simulink model "MCity_cs"  (Simulink 8.9)
settings: Solver=ode5  StartTime=0.0  StopTime=2.95  FixedStep=1/200  RelTol=1e-3
PreLoadFcn:
  | check_NUTS_defined;
  | 
  | assignin('base',['model_closed_' bdroot],false);
InitFcn:
  | PreScanExperimentInitFcn(bdroot)
StopFcn:
  | PreScanExperimentStopFcn(bdroot)
values from neighbouring files (symbols this model uses):
  d_offset = -18.15    [monocityTestLeftTurn.mat]    (also in simulation_leftTurn_PreScan.m = dl/vl*vh - 43 + R)
undefined symbols (not defined in the file or in its folder): DiscIntNeverNeededParam, warningInitialVelocity, x0
libraries: simulink x73, PreScanSimulinkLibrary x14, simulink_extras x10, PreScanUsefulBlocks x4
(part 4 of 11)

== system MCity_cs/TrafficLightDoubleUS_1/Traffic_Light On/Off  ==
  Range : Inport
  Compare To Constant : simulink/Logic and Bit Operations/Compare To Constant  relop=>=  const=1  OutDataTypeStr=uint8
  Constant : Constant
  Constant1 : Constant  Value=0
  Data Type Conversion{1,3..5} (4 alike) : DataTypeConversion
  Delay : Delay  DelayLength=40
  Logical Operator : Logic  Operator=NOT  AllPortsSameDT=off  OutDataTypeStr=boolean
  Logical Operator1 : Logic  Operator=NOT  AllPortsSameDT=off  OutDataTypeStr=boolean
  Logical Operator2 : Logic  Operator=NOT  AllPortsSameDT=off  OutDataTypeStr=boolean
  Logical Operator3 : Logic  AllPortsSameDT=off  OutDataTypeStr=boolean
  Logical Operator4 : Logic  AllPortsSameDT=off  OutDataTypeStr=boolean
  MinMax : MinMax  Function=max
  Pulse Generator : DiscretePulseGenerator  PulseType=Time based  Period=10  PulseWidth=50
  Switch{,1..3} (4 alike) : Switch  Criteria=u2 > Threshold
  Red : Outport
  Orange : Outport  Port=2
  Green : Outport  Port=3
  wires:
  Pulse Generator/1 -> Logical Operator1/1, Switch2/3
  Logical Operator1/1 -> Delay/1, Logical Operator3/2, Logical Operator4/1
  Delay/1 -> Logical Operator2/1, Logical Operator4/2
  Logical Operator2/1 -> Logical Operator3/1
  Logical Operator3/1 -> Data Type Conversion5/1
  Logical Operator4/1 -> Data Type Conversion4/1
  Constant/1 -> Switch/1
  Compare To Constant/1 -> Switch/2
  Constant1/1 -> Switch/3
  Switch/1 -> MinMax/1
  Logical Operator/1 -> Data Type Conversion3/1, Data Type Conversion1/1
  MinMax/1 -> Logical Operator/1, Switch1/2, Switch3/2, Switch2/1, Switch2/2
  Data Type Conversion1/1 -> Switch1/1
  Data Type Conversion4/1 -> Switch1/3
  Switch1/1 -> Red/1
  Data Type Conversion3/1 -> Switch3/1
  Switch3/1 -> Orange/1
  Data Type Conversion5/1 -> Switch3/3
  Switch2/1 -> Green/1
  Range/1 -> Compare To Constant/1

== system MCity_cs/TrafficLightDoubleUS_1/VISUCasingLights_1_Mux ==
  Red [-] : Inport
  Orange [-] : Inport  Port=2
  Green [-] : Inport  Port=3
  Mux1 : Mux  Inputs=3
  CasingLights : Outport
  wires:
  Green [-]/1 -> Mux1/3
  Mux1/1 -> CasingLights/1
  Orange [-]/1 -> Mux1/2
  Red [-]/1 -> Mux1/1

== system MCity_cs/TrafficLightDoubleUS_1/VISUCasingLights_2_Mux ==
  Red [-] : Inport
  Orange [-] : Inport  Port=2
  Green [-] : Inport  Port=3
  Mux1 : Mux  Inputs=3
  CasingLights : Outport
  wires:
  Green [-]/1 -> Mux1/3
  Mux1/1 -> CasingLights/1
  Orange [-]/1 -> Mux1/2
  Red [-]/1 -> Mux1/1

== system MCity_cs/TrafficLightDoubleUS_10/Perpendicular ==
  Compare To Constant : simulink/Logic and Bit Operations/Compare To Constant  relop=>=  const=1  OutDataTypeStr=uint8
  Constant : Constant
  Constant1 : Constant  Value=0
  Data Type Conversion{1,3..5} (4 alike) : DataTypeConversion
  Delay : Delay  DelayLength=40
  Ground_1 : Ground
  Logical Operator{,1..2,5} (4 alike) : Logic  Operator=NOT  AllPortsSameDT=off  OutDataTypeStr=boolean
  Logical Operator3 : Logic  AllPortsSameDT=off  OutDataTypeStr=boolean
  Logical Operator4 : Logic  AllPortsSameDT=off  OutDataTypeStr=boolean
  MinMax : MinMax  Function=max
  Pulse Generator : DiscretePulseGenerator  PulseType=Time based  Period=10  PulseWidth=50
  Switch{,1..3} (4 alike) : Switch  Criteria=u2 > Threshold
  Red : Outport
  Orange : Outport  Port=2
  Green : Outport  Port=3
  wires:
  Pulse Generator/1 -> Logical Operator5/1
  Logical Operator1/1 -> Delay/1, Logical Operator3/2, Logical Operator4/1
  Delay/1 -> Logical Operator2/1, Logical Operator4/2
  Logical Operator2/1 -> Logical Operator3/1
  Logical Operator3/1 -> Data Type Conversion5/1
  Logical Operator4/1 -> Data Type Conversion4/1
  Constant/1 -> Switch/1
  Compare To Constant/1 -> Switch/2
  Constant1/1 -> Switch/3
  Switch/1 -> MinMax/1
  Logical Operator/1 -> Data Type Conversion3/1, Data Type Conversion1/1
  MinMax/1 -> Logical Operator/1, Switch1/2, Switch3/2, Switch2/1, Switch2/2
  Data Type Conversion1/1 -> Switch1/1
  Data Type Conversion4/1 -> Switch1/3
  Switch1/1 -> Red/1
  Data Type Conversion3/1 -> Switch3/1
  Switch3/1 -> Orange/1
  Data Type Conversion5/1 -> Switch3/3
  Switch2/1 -> Green/1
  Logical Operator5/1 -> Logical Operator1/1, Switch2/3
  Ground_1/1 -> Compare To Constant/1

== system MCity_cs/TrafficLightDoubleUS_10/VISUCasingLights_1_Mux ==
  Red [-] : Inport
  Orange [-] : Inport  Port=2
  Green [-] : Inport  Port=3
  Mux1 : Mux  Inputs=3
  CasingLights : Outport
  wires:
  Green [-]/1 -> Mux1/3
  Mux1/1 -> CasingLights/1
  Orange [-]/1 -> Mux1/2
  Red [-]/1 -> Mux1/1

== system MCity_cs/TrafficLightDoubleUS_10/VISUCasingLights_2_Mux ==
  Red [-] : Inport
  Orange [-] : Inport  Port=2
  Green [-] : Inport  Port=3
  Mux1 : Mux  Inputs=3
  CasingLights : Outport
  wires:
  Green [-]/1 -> Mux1/3
  Mux1/1 -> CasingLights/1
  Orange [-]/1 -> Mux1/2
  Red [-]/1 -> Mux1/1

== system MCity_cs/TrafficLightDoubleUS_2/Traffic_Light On/Off  ==
  Range : Inport
  Compare To Constant : simulink/Logic and Bit Operations/Compare To Constant  relop=>=  const=1  OutDataTypeStr=uint8
  Constant : Constant
  Constant1 : Constant  Value=0
  Data Type Conversion{1,3..5} (4 alike) : DataTypeConversion
  Delay : Delay  DelayLength=40
  Logical Operator : Logic  Operator=NOT  AllPortsSameDT=off  OutDataTypeStr=boolean
  Logical Operator1 : Logic  Operator=NOT  AllPortsSameDT=off  OutDataTypeStr=boolean
  Logical Operator2 : Logic  Operator=NOT  AllPortsSameDT=off  OutDataTypeStr=boolean
  Logical Operator3 : Logic  AllPortsSameDT=off  OutDataTypeStr=boolean
  Logical Operator4 : Logic  AllPortsSameDT=off  OutDataTypeStr=boolean
  MinMax : MinMax  Function=max
  Pulse Generator : DiscretePulseGenerator  PulseType=Time based  Period=10  PulseWidth=50
  Switch{,1..3} (4 alike) : Switch  Criteria=u2 > Threshold
  Red : Outport
  Orange : Outport  Port=2
  Green : Outport  Port=3
  wires:
  Pulse Generator/1 -> Logical Operator1/1, Switch2/3
  Logical Operator1/1 -> Delay/1, Logical Operator3/2, Logical Operator4/1
  Delay/1 -> Logical Operator2/1, Logical Operator4/2
  Logical Operator2/1 -> Logical Operator3/1
  Logical Operator3/1 -> Data Type Conversion5/1
  Logical Operator4/1 -> Data Type Conversion4/1
  Constant/1 -> Switch/1
  Compare To Constant/1 -> Switch/2
  Constant1/1 -> Switch/3
  Switch/1 -> MinMax/1
  Logical Operator/1 -> Data Type Conversion3/1, Data Type Conversion1/1
  MinMax/1 -> Logical Operator/1, Switch1/2, Switch3/2, Switch2/1, Switch2/2
  Data Type Conversion1/1 -> Switch1/1
  Data Type Conversion4/1 -> Switch1/3
  Switch1/1 -> Red/1
  Data Type Conversion3/1 -> Switch3/1
  Switch3/1 -> Orange/1
  Data Type Conversion5/1 -> Switch3/3
  Switch2/1 -> Green/1
  Range/1 -> Compare To Constant/1

== system MCity_cs/TrafficLightDoubleUS_2/VISUCasingLights_1_Mux ==
  Red [-] : Inport
  Orange [-] : Inport  Port=2
  Green [-] : Inport  Port=3
  Mux1 : Mux  Inputs=3
  CasingLights : Outport
  wires:
  Green [-]/1 -> Mux1/3
  Mux1/1 -> CasingLights/1
  Orange [-]/1 -> Mux1/2
  Red [-]/1 -> Mux1/1

== system MCity_cs/TrafficLightDoubleUS_2/VISUCasingLights_2_Mux ==
  Red [-] : Inport
  Orange [-] : Inport  Port=2
  Green [-] : Inport  Port=3
  Mux1 : Mux  Inputs=3
  CasingLights : Outport
  wires:
  Green [-]/1 -> Mux1/3
  Mux1/1 -> CasingLights/1
  Orange [-]/1 -> Mux1/2
  Red [-]/1 -> Mux1/1

== system MCity_cs/TrafficLightDoubleUS_3/Perpendicular ==
  Compare To Constant : simulink/Logic and Bit Operations/Compare To Constant  relop=>=  const=1  OutDataTypeStr=uint8
  Constant : Constant
  Constant1 : Constant  Value=0
  Constant2 : Constant  Value=0
  Data Type Conversion{1,3..5} (4 alike) : DataTypeConversion
  Delay : Delay  DelayLength=40
  Ground_1 : Ground
  Ground_2 : Ground
  Logical Operator : Logic  Operator=NOT  AllPortsSameDT=off  OutDataTypeStr=boolean
  Logical Operator1 : Logic  Operator=NOT  AllPortsSameDT=off  OutDataTypeStr=boolean
  Logical Operator2 : Logic  Operator=NOT  AllPortsSameDT=off  OutDataTypeStr=boolean
  Logical Operator3 : Logic  AllPortsSameDT=off  OutDataTypeStr=boolean
  Logical Operator4 : Logic  AllPortsSameDT=off  OutDataTypeStr=boolean
  MinMax : MinMax  Function=max
  Switch{,1..3} (4 alike) : Switch  Criteria=u2 > Threshold
  Terminator_1 : Terminator
  Red : Outport
  Orange : Outport  Port=2
  Green : Outport  Port=3
  wires:
  Constant2/1 -> Logical Operator1/1, Switch2/3
  Logical Operator1/1 -> Delay/1, Logical Operator3/2, Logical Operator4/1
  Delay/1 -> Logical Operator2/1, Logical Operator4/2
  Logical Operator2/1 -> Logical Operator3/1
  Logical Operator3/1 -> Data Type Conversion5/1
  Logical Operator4/1 -> Data Type Conversion4/1
  Constant/1 -> Switch/1
  Constant1/1 -> Switch/3
  Switch/1 -> MinMax/1
  Logical Operator/1 -> Data Type Conversion3/1, Data Type Conversion1/1
  MinMax/1 -> Logical Operator/1, Switch1/2, Switch3/2, Switch2/1, Switch2/2
  Data Type Conversion1/1 -> Switch1/1
  Data Type Conversion4/1 -> Switch1/3
  Switch1/1 -> Red/1
  Data Type Conversion3/1 -> Switch3/1
  Switch3/1 -> Orange/1
  Data Type Conversion5/1 -> Switch3/3
  Switch2/1 -> Green/1
  Ground_1/1 -> Compare To Constant/1
  Compare To Constant/1 -> Terminator_1/1
  Ground_2/1 -> Switch/2

== system MCity_cs/TrafficLightDoubleUS_3/VISUCasingLights_1_Mux ==
  Red [-] : Inport
  Orange [-] : Inport  Port=2
  Green [-] : Inport  Port=3
  Mux1 : Mux  Inputs=3
  CasingLights : Outport
  wires:
  Green [-]/1 -> Mux1/3
  Mux1/1 -> CasingLights/1
  Orange [-]/1 -> Mux1/2
  Red [-]/1 -> Mux1/1

== system MCity_cs/TrafficLightDoubleUS_3/VISUCasingLights_2_Mux ==
  Red [-] : Inport
  Orange [-] : Inport  Port=2
  Green [-] : Inport  Port=3
  Mux1 : Mux  Inputs=3
  CasingLights : Outport
  wires:
  Green [-]/1 -> Mux1/3
  Mux1/1 -> CasingLights/1
  Orange [-]/1 -> Mux1/2
  Red [-]/1 -> Mux1/1

== system MCity_cs/TrafficLightDoubleUS_4/Perpendicular ==
  Compare To Constant : simulink/Logic and Bit Operations/Compare To Constant  relop=>=  const=1  OutDataTypeStr=uint8
  Constant : Constant
  Constant1 : Constant  Value=0
  Data Type Conversion{1,3..5} (4 alike) : DataTypeConversion
  Delay : Delay  DelayLength=40
  Ground_1 : Ground
  Logical Operator{,1..2,5} (4 alike) : Logic  Operator=NOT  AllPortsSameDT=off  OutDataTypeStr=boolean
  Logical Operator3 : Logic  AllPortsSameDT=off  OutDataTypeStr=boolean
  Logical Operator4 : Logic  AllPortsSameDT=off  OutDataTypeStr=boolean
  MinMax : MinMax  Function=max
  Pulse Generator : DiscretePulseGenerator  PulseType=Time based  Period=10  PulseWidth=50
  Switch{,1..3} (4 alike) : Switch  Criteria=u2 > Threshold
  Red : Outport
  Orange : Outport  Port=2
  Green : Outport  Port=3
  wires:
  Pulse Generator/1 -> Logical Operator5/1
  Logical Operator1/1 -> Delay/1, Logical Operator3/2, Logical Operator4/1
  Delay/1 -> Logical Operator2/1, Logical Operator4/2
  Logical Operator2/1 -> Logical Operator3/1
  Logical Operator3/1 -> Data Type Conversion5/1
  Logical Operator4/1 -> Data Type Conversion4/1
  Constant/1 -> Switch/1
  Compare To Constant/1 -> Switch/2
  Constant1/1 -> Switch/3
  Switch/1 -> MinMax/1
  Logical Operator/1 -> Data Type Conversion3/1, Data Type Conversion1/1
  MinMax/1 -> Logical Operator/1, Switch1/2, Switch3/2, Switch2/1, Switch2/2
  Data Type Conversion1/1 -> Switch1/1
  Data Type Conversion4/1 -> Switch1/3
  Switch1/1 -> Red/1
  Data Type Conversion3/1 -> Switch3/1
  Switch3/1 -> Orange/1
  Data Type Conversion5/1 -> Switch3/3
  Switch2/1 -> Green/1
  Logical Operator5/1 -> Logical Operator1/1, Switch2/3
  Ground_1/1 -> Compare To Constant/1

== system MCity_cs/TrafficLightDoubleUS_4/VISUCasingLights_1_Mux ==
  Red [-] : Inport
  Orange [-] : Inport  Port=2
  Green [-] : Inport  Port=3
  Mux1 : Mux  Inputs=3
  CasingLights : Outport
  wires:
  Green [-]/1 -> Mux1/3
  Mux1/1 -> CasingLights/1
  Orange [-]/1 -> Mux1/2
  Red [-]/1 -> Mux1/1

== system MCity_cs/TrafficLightDoubleUS_4/VISUCasingLights_2_Mux ==
  Red [-] : Inport
  Orange [-] : Inport  Port=2
  Green [-] : Inport  Port=3
  Mux1 : Mux  Inputs=3
  CasingLights : Outport
  wires:
  Green [-]/1 -> Mux1/3
  Mux1/1 -> CasingLights/1
  Orange [-]/1 -> Mux1/2
  Red [-]/1 -> Mux1/1

== system MCity_cs/TrafficLightDoubleUS_7/Traffic_Light On/Off  ==
  Range : Inport
  Compare To Constant : simulink/Logic and Bit Operations/Compare To Constant  relop=>=  const=1  OutDataTypeStr=uint8
  Constant : Constant
  Constant1 : Constant  Value=0
  Data Type Conversion{1,3..5} (4 alike) : DataTypeConversion
  Delay : Delay  DelayLength=40
  Logical Operator : Logic  Operator=NOT  AllPortsSameDT=off  OutDataTypeStr=boolean
  Logical Operator1 : Logic  Operator=NOT  AllPortsSameDT=off  OutDataTypeStr=boolean
  Logical Operator2 : Logic  Operator=NOT  AllPortsSameDT=off  OutDataTypeStr=boolean
  Logical Operator3 : Logic  AllPortsSameDT=off  OutDataTypeStr=boolean
  Logical Operator4 : Logic  AllPortsSameDT=off  OutDataTypeStr=boolean
  MinMax : MinMax  Function=max
  Pulse Generator : DiscretePulseGenerator  PulseType=Time based  Period=10  PulseWidth=50
  Switch{,1..3} (4 alike) : Switch  Criteria=u2 > Threshold
  Red : Outport
  Orange : Outport  Port=2
  Green : Outport  Port=3
  wires:
  Pulse Generator/1 -> Logical Operator1/1, Switch2/3
  Logical Operator1/1 -> Delay/1, Logical Operator3/2, Logical Operator4/1
  Delay/1 -> Logical Operator2/1, Logical Operator4/2
  Logical Operator2/1 -> Logical Operator3/1
  Logical Operator3/1 -> Data Type Conversion5/1
  Logical Operator4/1 -> Data Type Conversion4/1
  Constant/1 -> Switch/1
  Compare To Constant/1 -> Switch/2
  Constant1/1 -> Switch/3
  Switch/1 -> MinMax/1
  Logical Operator/1 -> Data Type Conversion3/1, Data Type Conversion1/1
  MinMax/1 -> Logical Operator/1, Switch1/2, Switch3/2, Switch2/1, Switch2/2
  Data Type Conversion1/1 -> Switch1/1
  Data Type Conversion4/1 -> Switch1/3
  Switch1/1 -> Red/1
  Data Type Conversion3/1 -> Switch3/1
  Switch3/1 -> Orange/1
  Data Type Conversion5/1 -> Switch3/3
  Switch2/1 -> Green/1
  Range/1 -> Compare To Constant/1

== system MCity_cs/TrafficLightDoubleUS_7/VISUCasingLights_1_Mux ==
  Red [-] : Inport
  Orange [-] : Inport  Port=2
  Green [-] : Inport  Port=3
  Mux1 : Mux  Inputs=3
  CasingLights : Outport
  wires:
  Green [-]/1 -> Mux1/3
  Mux1/1 -> CasingLights/1
  Orange [-]/1 -> Mux1/2
  Red [-]/1 -> Mux1/1

== system MCity_cs/TrafficLightDoubleUS_7/VISUCasingLights_2_Mux ==
  Red [-] : Inport
  Orange [-] : Inport  Port=2
  Green [-] : Inport  Port=3
  Mux1 : Mux  Inputs=3
  CasingLights : Outport
  wires:
  Green [-]/1 -> Mux1/3
  Mux1/1 -> CasingLights/1
  Orange [-]/1 -> Mux1/2
  Red [-]/1 -> Mux1/1

== system MCity_cs/TrafficLightDoubleUS_8/Traffic_Light On/Off  ==
  Range : Inport
  Compare To Constant : simulink/Logic and Bit Operations/Compare To Constant  relop=>=  const=1  OutDataTypeStr=uint8
  Constant : Constant
  Constant1 : Constant  Value=0
  Data Type Conversion{1,3..5} (4 alike) : DataTypeConversion
  Delay : Delay  DelayLength=40
  Logical Operator : Logic  Operator=NOT  AllPortsSameDT=off  OutDataTypeStr=boolean
  Logical Operator1 : Logic  Operator=NOT  AllPortsSameDT=off  OutDataTypeStr=boolean
  Logical Operator2 : Logic  Operator=NOT  AllPortsSameDT=off  OutDataTypeStr=boolean
  Logical Operator3 : Logic  AllPortsSameDT=off  OutDataTypeStr=boolean
  Logical Operator4 : Logic  AllPortsSameDT=off  OutDataTypeStr=boolean
  MinMax : MinMax  Function=max
  Pulse Generator : DiscretePulseGenerator  PulseType=Time based  Period=10  PulseWidth=50
  Switch{,1..3} (4 alike) : Switch  Criteria=u2 > Threshold
  Red : Outport
  Orange : Outport  Port=2
  Green : Outport  Port=3
  wires:
  Pulse Generator/1 -> Logical Operator1/1, Switch2/3
  Logical Operator1/1 -> Delay/1, Logical Operator3/2, Logical Operator4/1
  Delay/1 -> Logical Operator2/1, Logical Operator4/2
  Logical Operator2/1 -> Logical Operator3/1
  Logical Operator3/1 -> Data Type Conversion5/1
  Logical Operator4/1 -> Data Type Conversion4/1
  Constant/1 -> Switch/1
  Compare To Constant/1 -> Switch/2
  Constant1/1 -> Switch/3
  Switch/1 -> MinMax/1
  Logical Operator/1 -> Data Type Conversion3/1, Data Type Conversion1/1
  MinMax/1 -> Logical Operator/1, Switch1/2, Switch3/2, Switch2/1, Switch2/2
  Data Type Conversion1/1 -> Switch1/1
  Data Type Conversion4/1 -> Switch1/3
  Switch1/1 -> Red/1
  Data Type Conversion3/1 -> Switch3/1
  Switch3/1 -> Orange/1
  Data Type Conversion5/1 -> Switch3/3
  Switch2/1 -> Green/1
  Range/1 -> Compare To Constant/1

== system MCity_cs/TrafficLightDoubleUS_8/VISUCasingLights_1_Mux ==
  Red [-] : Inport
  Orange [-] : Inport  Port=2
  Green [-] : Inport  Port=3
  Mux1 : Mux  Inputs=3
  CasingLights : Outport
  wires:
  Green [-]/1 -> Mux1/3
  Mux1/1 -> CasingLights/1
  Orange [-]/1 -> Mux1/2
  Red [-]/1 -> Mux1/1

== system MCity_cs/TrafficLightDoubleUS_8/VISUCasingLights_2_Mux ==
  Red [-] : Inport
  Orange [-] : Inport  Port=2
  Green [-] : Inport  Port=3
  Mux1 : Mux  Inputs=3
  CasingLights : Outport
  wires:
  Green [-]/1 -> Mux1/3
  Mux1/1 -> CasingLights/1
  Orange [-]/1 -> Mux1/2
  Red [-]/1 -> Mux1/1

== system MCity_cs/TrafficLightDoubleUS_9/Traffic_Light On/Off  ==
  Range : Inport
  Compare To Constant : simulink/Logic and Bit Operations/Compare To Constant  relop=>=  const=1  OutDataTypeStr=uint8
  Constant : Constant
  Constant1 : Constant  Value=0
  Data Type Conversion{1,3..5} (4 alike) : DataTypeConversion
  Delay : Delay  DelayLength=40
  Logical Operator : Logic  Operator=NOT  AllPortsSameDT=off  OutDataTypeStr=boolean
  Logical Operator1 : Logic  Operator=NOT  AllPortsSameDT=off  OutDataTypeStr=boolean
  Logical Operator2 : Logic  Operator=NOT  AllPortsSameDT=off  OutDataTypeStr=boolean
  Logical Operator3 : Logic  AllPortsSameDT=off  OutDataTypeStr=boolean
  Logical Operator4 : Logic  AllPortsSameDT=off  OutDataTypeStr=boolean
  MinMax : MinMax  Function=max
  Pulse Generator : DiscretePulseGenerator  PulseType=Time based  Period=10  PulseWidth=50
  Switch{,1..3} (4 alike) : Switch  Criteria=u2 > Threshold
  Red : Outport
  Orange : Outport  Port=2
  Green : Outport  Port=3
  wires:
  Pulse Generator/1 -> Logical Operator1/1, Switch2/3
  Logical Operator1/1 -> Delay/1, Logical Operator3/2, Logical Operator4/1
  Delay/1 -> Logical Operator2/1, Logical Operator4/2
  Logical Operator2/1 -> Logical Operator3/1
  Logical Operator3/1 -> Data Type Conversion5/1
  Logical Operator4/1 -> Data Type Conversion4/1
  Constant/1 -> Switch/1
  Compare To Constant/1 -> Switch/2
  Constant1/1 -> Switch/3
  Switch/1 -> MinMax/1
  Logical Operator/1 -> Data Type Conversion3/1, Data Type Conversion1/1
  MinMax/1 -> Logical Operator/1, Switch1/2, Switch3/2, Switch2/1, Switch2/2
  Data Type Conversion1/1 -> Switch1/1
  Data Type Conversion4/1 -> Switch1/3
  Switch1/1 -> Red/1
  Data Type Conversion3/1 -> Switch3/1
  Switch3/1 -> Orange/1
  Data Type Conversion5/1 -> Switch3/3
  Switch2/1 -> Green/1
  Range/1 -> Compare To Constant/1

== system MCity_cs/TrafficLightDoubleUS_9/VISUCasingLights_1_Mux ==
  Red [-] : Inport
  Orange [-] : Inport  Port=2
  Green [-] : Inport  Port=3
  Mux1 : Mux  Inputs=3
  CasingLights : Outport
  wires:
  Green [-]/1 -> Mux1/3
  Mux1/1 -> CasingLights/1
  Orange [-]/1 -> Mux1/2
  Red [-]/1 -> Mux1/1

== system MCity_cs/TrafficLightDoubleUS_9/VISUCasingLights_2_Mux ==
  Red [-] : Inport
  Orange [-] : Inport  Port=2
  Green [-] : Inport  Port=3
  Mux1 : Mux  Inputs=3
  CasingLights : Outport
  wires:
  Green [-]/1 -> Mux1/3
  Mux1/1 -> CasingLights/1
  Orange [-]/1 -> Mux1/2
  Red [-]/1 -> Mux1/1

== system MCity_cs/VISUCasingLights_1_TrafficLightDoubleUS_1/conv_Green ==
  on_off : Inport
  Constant5 : Constant  Value=[5 32 25 255 0 64 50 255 0 64 50 255 0 0 0 255]
  Constant9 : Constant  Value="[0 45 34 255  0 45 34 255  0 45 34 255  30 306 240 255]"
  Switch2 : Switch  Threshold=0.5
  RGBcolor : Outport
  wires:
  Switch2/1 -> RGBcolor/1
  on_off/1 -> Switch2/2
  Constant5/1 -> Switch2/3  "off"
  Constant9/1 -> Switch2/1  "on"

== system MCity_cs/VISUCasingLights_1_TrafficLightDoubleUS_1/conv_Orange ==
  on_off : Inport
  Constant2 : Constant  Value="[45 34 0 255  45 34 0 255  45 34 0 255  306 229 5 255]"
  Constant20 : Constant  Value=[32 25 5 255 64 48 5 255 64 54 5 255 0 0 0 255]
  Switch1 : Switch  Threshold=0.5
  RGBcolor : Outport
  wires:
  Constant20/1 -> Switch1/3  "off"
  Constant2/1 -> Switch1/1  "on"
  on_off/1 -> Switch1/2
  Switch1/1 -> RGBcolor/1

== system MCity_cs/VISUCasingLights_1_TrafficLightDoubleUS_1/conv_Red ==
  on_off : Inport
  Constant2 : Constant  Value="[45 0 0 255  45 0 0 255  45 0 0 255 306 30 30 255]"
  Constant20 : Constant  Value=[32 5 5 255 64 5 5 255 64 5 5 255 0 0 0 255]
  Switch1 : Switch  Threshold=0.5
  RGBcolor : Outport
  wires:
  Constant20/1 -> Switch1/3  "off"
  Constant2/1 -> Switch1/1  "on"
  on_off/1 -> Switch1/2
  Switch1/1 -> RGBcolor/1

== system MCity_cs/VISUCasingLights_1_TrafficLightDoubleUS_1/visu_CasingGreen ==
  Y : Inport
  Assignment : Assignment  IndexMode=Zero-based  SampleTime=TimeStep  IndexOptions=Starting index (dialog)  Indices=PortIndex  OutputSizes=[1 1]
  Data Store Read : DataStoreRead  DataStoreName=SimCoreActuators  SampleTime=TimeStep
  Data Store Write : DataStoreWrite  DataStoreName=SimCoreActuators
  wires:
  Assignment/1 -> Data Store Write/1
  Data Store Read/1 -> Assignment/1
  Y/1 -> Assignment/2

== system MCity_cs/VISUCasingLights_1_TrafficLightDoubleUS_1/visu_CasingOrange ==
  Y : Inport
  Assignment : Assignment  IndexMode=Zero-based  SampleTime=TimeStep  IndexOptions=Starting index (dialog)  Indices=PortIndex  OutputSizes=[1 1]
  Data Store Read : DataStoreRead  DataStoreName=SimCoreActuators  SampleTime=TimeStep
  Data Store Write : DataStoreWrite  DataStoreName=SimCoreActuators
  wires:
  Assignment/1 -> Data Store Write/1
  Data Store Read/1 -> Assignment/1
  Y/1 -> Assignment/2

== system MCity_cs/VISUCasingLights_1_TrafficLightDoubleUS_1/visu_CasingRed ==
  Y : Inport
  Assignment : Assignment  IndexMode=Zero-based  SampleTime=TimeStep  IndexOptions=Starting index (dialog)  Indices=PortIndex  OutputSizes=[1 1]
  Data Store Read : DataStoreRead  DataStoreName=SimCoreActuators  SampleTime=TimeStep
  Data Store Write : DataStoreWrite  DataStoreName=SimCoreActuators
  wires:
  Assignment/1 -> Data Store Write/1
  Data Store Read/1 -> Assignment/1
  Y/1 -> Assignment/2

== system MCity_cs/VISUCasingLights_1_TrafficLightDoubleUS_10/conv_Green ==
  on_off : Inport
  Constant5 : Constant  Value=[5 32 25 255 0 64 50 255 0 64 50 255 0 0 0 255]
  Constant9 : Constant  Value="[0 45 34 255  0 45 34 255  0 45 34 255  30 306 240 255]"
  Switch2 : Switch  Threshold=0.5
  RGBcolor : Outport
  wires:
  Switch2/1 -> RGBcolor/1
  on_off/1 -> Switch2/2
  Constant5/1 -> Switch2/3  "off"
  Constant9/1 -> Switch2/1  "on"

== system MCity_cs/VISUCasingLights_1_TrafficLightDoubleUS_10/conv_Orange ==
  on_off : Inport
  Constant2 : Constant  Value="[45 34 0 255  45 34 0 255  45 34 0 255  306 229 5 255]"
  Constant20 : Constant  Value=[32 25 5 255 64 48 5 255 64 54 5 255 0 0 0 255]
  Switch1 : Switch  Threshold=0.5
  RGBcolor : Outport
  wires:
  Constant20/1 -> Switch1/3  "off"
  Constant2/1 -> Switch1/1  "on"
  on_off/1 -> Switch1/2
  Switch1/1 -> RGBcolor/1

== system MCity_cs/VISUCasingLights_1_TrafficLightDoubleUS_10/conv_Red ==
  on_off : Inport
  Constant2 : Constant  Value="[45 0 0 255  45 0 0 255  45 0 0 255 306 30 30 255]"
  Constant20 : Constant  Value=[32 5 5 255 64 5 5 255 64 5 5 255 0 0 0 255]
  Switch1 : Switch  Threshold=0.5
  RGBcolor : Outport
  wires:
  Constant20/1 -> Switch1/3  "off"
  Constant2/1 -> Switch1/1  "on"
  on_off/1 -> Switch1/2
  Switch1/1 -> RGBcolor/1

== system MCity_cs/VISUCasingLights_1_TrafficLightDoubleUS_10/visu_CasingGreen ==
  Y : Inport
  Assignment : Assignment  IndexMode=Zero-based  SampleTime=TimeStep  IndexOptions=Starting index (dialog)  Indices=PortIndex  OutputSizes=[1 1]
  Data Store Read : DataStoreRead  DataStoreName=SimCoreActuators  SampleTime=TimeStep
  Data Store Write : DataStoreWrite  DataStoreName=SimCoreActuators
  wires:
  Assignment/1 -> Data Store Write/1
  Data Store Read/1 -> Assignment/1
  Y/1 -> Assignment/2

== system MCity_cs/VISUCasingLights_1_TrafficLightDoubleUS_10/visu_CasingOrange ==
  Y : Inport
  Assignment : Assignment  IndexMode=Zero-based  SampleTime=TimeStep  IndexOptions=Starting index (dialog)  Indices=PortIndex  OutputSizes=[1 1]
  Data Store Read : DataStoreRead  DataStoreName=SimCoreActuators  SampleTime=TimeStep
  Data Store Write : DataStoreWrite  DataStoreName=SimCoreActuators
  wires:
  Assignment/1 -> Data Store Write/1
  Data Store Read/1 -> Assignment/1
  Y/1 -> Assignment/2

== system MCity_cs/VISUCasingLights_1_TrafficLightDoubleUS_10/visu_CasingRed ==
  Y : Inport
  Assignment : Assignment  IndexMode=Zero-based  SampleTime=TimeStep  IndexOptions=Starting index (dialog)  Indices=PortIndex  OutputSizes=[1 1]
  Data Store Read : DataStoreRead  DataStoreName=SimCoreActuators  SampleTime=TimeStep
  Data Store Write : DataStoreWrite  DataStoreName=SimCoreActuators
  wires:
  Assignment/1 -> Data Store Write/1
  Data Store Read/1 -> Assignment/1
  Y/1 -> Assignment/2

== system MCity_cs/VISUCasingLights_1_TrafficLightDoubleUS_2/conv_Green ==
  on_off : Inport
  Constant5 : Constant  Value=[5 32 25 255 0 64 50 255 0 64 50 255 0 0 0 255]
  Constant9 : Constant  Value="[0 45 34 255  0 45 34 255  0 45 34 255  30 306 240 255]"
  Switch2 : Switch  Threshold=0.5
  RGBcolor : Outport
  wires:
  Switch2/1 -> RGBcolor/1
  on_off/1 -> Switch2/2
  Constant5/1 -> Switch2/3  "off"
  Constant9/1 -> Switch2/1  "on"

== system MCity_cs/VISUCasingLights_1_TrafficLightDoubleUS_2/conv_Orange ==
  on_off : Inport
  Constant2 : Constant  Value="[45 34 0 255  45 34 0 255  45 34 0 255  306 229 5 255]"
  Constant20 : Constant  Value=[32 25 5 255 64 48 5 255 64 54 5 255 0 0 0 255]
  Switch1 : Switch  Threshold=0.5
  RGBcolor : Outport
  wires:
  Constant20/1 -> Switch1/3  "off"
  Constant2/1 -> Switch1/1  "on"
  on_off/1 -> Switch1/2
  Switch1/1 -> RGBcolor/1

== system MCity_cs/VISUCasingLights_1_TrafficLightDoubleUS_2/conv_Red ==
  on_off : Inport
  Constant2 : Constant  Value="[45 0 0 255  45 0 0 255  45 0 0 255 306 30 30 255]"
  Constant20 : Constant  Value=[32 5 5 255 64 5 5 255 64 5 5 255 0 0 0 255]
  Switch1 : Switch  Threshold=0.5
  RGBcolor : Outport
  wires:
  Constant20/1 -> Switch1/3  "off"
  Constant2/1 -> Switch1/1  "on"
  on_off/1 -> Switch1/2
  Switch1/1 -> RGBcolor/1

== system MCity_cs/VISUCasingLights_1_TrafficLightDoubleUS_2/visu_CasingGreen ==
  Y : Inport
  Assignment : Assignment  IndexMode=Zero-based  SampleTime=TimeStep  IndexOptions=Starting index (dialog)  Indices=PortIndex  OutputSizes=[1 1]
  Data Store Read : DataStoreRead  DataStoreName=SimCoreActuators  SampleTime=TimeStep
  Data Store Write : DataStoreWrite  DataStoreName=SimCoreActuators
  wires:
  Assignment/1 -> Data Store Write/1
  Data Store Read/1 -> Assignment/1
  Y/1 -> Assignment/2

== system MCity_cs/VISUCasingLights_1_TrafficLightDoubleUS_2/visu_CasingOrange ==
  Y : Inport
  Assignment : Assignment  IndexMode=Zero-based  SampleTime=TimeStep  IndexOptions=Starting index (dialog)  Indices=PortIndex  OutputSizes=[1 1]
  Data Store Read : DataStoreRead  DataStoreName=SimCoreActuators  SampleTime=TimeStep
  Data Store Write : DataStoreWrite  DataStoreName=SimCoreActuators
  wires:
  Assignment/1 -> Data Store Write/1
  Data Store Read/1 -> Assignment/1
  Y/1 -> Assignment/2

== system MCity_cs/VISUCasingLights_1_TrafficLightDoubleUS_2/visu_CasingRed ==
  Y : Inport
  Assignment : Assignment  IndexMode=Zero-based  SampleTime=TimeStep  IndexOptions=Starting index (dialog)  Indices=PortIndex  OutputSizes=[1 1]
  Data Store Read : DataStoreRead  DataStoreName=SimCoreActuators  SampleTime=TimeStep
  Data Store Write : DataStoreWrite  DataStoreName=SimCoreActuators
  wires:
  Assignment/1 -> Data Store Write/1
  Data Store Read/1 -> Assignment/1
  Y/1 -> Assignment/2

== system MCity_cs/VISUCasingLights_1_TrafficLightDoubleUS_3/conv_Green ==
  on_off : Inport
  Constant5 : Constant  Value=[5 32 25 255 0 64 50 255 0 64 50 255 0 0 0 255]
  Constant9 : Constant  Value="[0 45 34 255  0 45 34 255  0 45 34 255  30 306 240 255]"
  Switch2 : Switch  Threshold=0.5
  RGBcolor : Outport
  wires:
  Switch2/1 -> RGBcolor/1
  on_off/1 -> Switch2/2
  Constant5/1 -> Switch2/3  "off"
  Constant9/1 -> Switch2/1  "on"

== system MCity_cs/VISUCasingLights_1_TrafficLightDoubleUS_3/conv_Orange ==
  on_off : Inport
  Constant2 : Constant  Value="[45 34 0 255  45 34 0 255  45 34 0 255  306 229 5 255]"
  Constant20 : Constant  Value=[32 25 5 255 64 48 5 255 64 54 5 255 0 0 0 255]
  Switch1 : Switch  Threshold=0.5
  RGBcolor : Outport
  wires:
  Constant20/1 -> Switch1/3  "off"
  Constant2/1 -> Switch1/1  "on"
  on_off/1 -> Switch1/2
  Switch1/1 -> RGBcolor/1

== system MCity_cs/VISUCasingLights_1_TrafficLightDoubleUS_3/conv_Red ==
  on_off : Inport
  Constant2 : Constant  Value="[45 0 0 255  45 0 0 255  45 0 0 255 306 30 30 255]"
  Constant20 : Constant  Value=[32 5 5 255 64 5 5 255 64 5 5 255 0 0 0 255]
  Switch1 : Switch  Threshold=0.5
  RGBcolor : Outport
  wires:
  Constant20/1 -> Switch1/3  "off"
  Constant2/1 -> Switch1/1  "on"
  on_off/1 -> Switch1/2
  Switch1/1 -> RGBcolor/1

== system MCity_cs/VISUCasingLights_1_TrafficLightDoubleUS_3/visu_CasingGreen ==
  Y : Inport
  Assignment : Assignment  IndexMode=Zero-based  SampleTime=TimeStep  IndexOptions=Starting index (dialog)  Indices=PortIndex  OutputSizes=[1 1]
  Data Store Read : DataStoreRead  DataStoreName=SimCoreActuators  SampleTime=TimeStep
  Data Store Write : DataStoreWrite  DataStoreName=SimCoreActuators
  wires:
  Assignment/1 -> Data Store Write/1
  Data Store Read/1 -> Assignment/1
  Y/1 -> Assignment/2

== system MCity_cs/VISUCasingLights_1_TrafficLightDoubleUS_3/visu_CasingOrange ==
  Y : Inport
  Assignment : Assignment  IndexMode=Zero-based  SampleTime=TimeStep  IndexOptions=Starting index (dialog)  Indices=PortIndex  OutputSizes=[1 1]
  Data Store Read : DataStoreRead  DataStoreName=SimCoreActuators  SampleTime=TimeStep
  Data Store Write : DataStoreWrite  DataStoreName=SimCoreActuators
  wires:
  Assignment/1 -> Data Store Write/1
  Data Store Read/1 -> Assignment/1
  Y/1 -> Assignment/2

== system MCity_cs/VISUCasingLights_1_TrafficLightDoubleUS_3/visu_CasingRed ==
  Y : Inport
  Assignment : Assignment  IndexMode=Zero-based  SampleTime=TimeStep  IndexOptions=Starting index (dialog)  Indices=PortIndex  OutputSizes=[1 1]
  Data Store Read : DataStoreRead  DataStoreName=SimCoreActuators  SampleTime=TimeStep
  Data Store Write : DataStoreWrite  DataStoreName=SimCoreActuators
  wires:
  Assignment/1 -> Data Store Write/1
  Data Store Read/1 -> Assignment/1
  Y/1 -> Assignment/2

== system MCity_cs/VISUCasingLights_1_TrafficLightDoubleUS_4/conv_Green ==
  on_off : Inport
  Constant5 : Constant  Value=[5 32 25 255 0 64 50 255 0 64 50 255 0 0 0 255]
  Constant9 : Constant  Value="[0 45 34 255  0 45 34 255  0 45 34 255  30 306 240 255]"
  Switch2 : Switch  Threshold=0.5
  RGBcolor : Outport
  wires:
  Switch2/1 -> RGBcolor/1
  on_off/1 -> Switch2/2
  Constant5/1 -> Switch2/3  "off"
  Constant9/1 -> Switch2/1  "on"

== system MCity_cs/VISUCasingLights_1_TrafficLightDoubleUS_4/conv_Orange ==
  on_off : Inport
  Constant2 : Constant  Value="[45 34 0 255  45 34 0 255  45 34 0 255  306 229 5 255]"
  Constant20 : Constant  Value=[32 25 5 255 64 48 5 255 64 54 5 255 0 0 0 255]
  Switch1 : Switch  Threshold=0.5
  RGBcolor : Outport
  wires:
  Constant20/1 -> Switch1/3  "off"
  Constant2/1 -> Switch1/1  "on"
  on_off/1 -> Switch1/2
  Switch1/1 -> RGBcolor/1

== system MCity_cs/VISUCasingLights_1_TrafficLightDoubleUS_4/conv_Red ==
  on_off : Inport
  Constant2 : Constant  Value="[45 0 0 255  45 0 0 255  45 0 0 255 306 30 30 255]"
  Constant20 : Constant  Value=[32 5 5 255 64 5 5 255 64 5 5 255 0 0 0 255]
  Switch1 : Switch  Threshold=0.5
  RGBcolor : Outport
  wires:
  Constant20/1 -> Switch1/3  "off"
  Constant2/1 -> Switch1/1  "on"
  on_off/1 -> Switch1/2
  Switch1/1 -> RGBcolor/1

== system MCity_cs/VISUCasingLights_1_TrafficLightDoubleUS_4/visu_CasingGreen ==
  Y : Inport
  Assignment : Assignment  IndexMode=Zero-based  SampleTime=TimeStep  IndexOptions=Starting index (dialog)  Indices=PortIndex  OutputSizes=[1 1]
  Data Store Read : DataStoreRead  DataStoreName=SimCoreActuators  SampleTime=TimeStep
  Data Store Write : DataStoreWrite  DataStoreName=SimCoreActuators
  wires:
  Assignment/1 -> Data Store Write/1
  Data Store Read/1 -> Assignment/1
  Y/1 -> Assignment/2

== system MCity_cs/VISUCasingLights_1_TrafficLightDoubleUS_4/visu_CasingOrange ==
  Y : Inport
  Assignment : Assignment  IndexMode=Zero-based  SampleTime=TimeStep  IndexOptions=Starting index (dialog)  Indices=PortIndex  OutputSizes=[1 1]
  Data Store Read : DataStoreRead  DataStoreName=SimCoreActuators  SampleTime=TimeStep
  Data Store Write : DataStoreWrite  DataStoreName=SimCoreActuators
  wires:
  Assignment/1 -> Data Store Write/1
  Data Store Read/1 -> Assignment/1
  Y/1 -> Assignment/2

== system MCity_cs/VISUCasingLights_1_TrafficLightDoubleUS_4/visu_CasingRed ==
  Y : Inport
  Assignment : Assignment  IndexMode=Zero-based  SampleTime=TimeStep  IndexOptions=Starting index (dialog)  Indices=PortIndex  OutputSizes=[1 1]
  Data Store Read : DataStoreRead  DataStoreName=SimCoreActuators  SampleTime=TimeStep
  Data Store Write : DataStoreWrite  DataStoreName=SimCoreActuators
  wires:
  Assignment/1 -> Data Store Write/1
  Data Store Read/1 -> Assignment/1
  Y/1 -> Assignment/2

== system MCity_cs/VISUCasingLights_1_TrafficLightDoubleUS_7/conv_Green ==
  on_off : Inport
  Constant5 : Constant  Value=[5 32 25 255 0 64 50 255 0 64 50 255 0 0 0 255]
  Constant9 : Constant  Value="[0 45 34 255  0 45 34 255  0 45 34 255  30 306 240 255]"
  Switch2 : Switch  Threshold=0.5
  RGBcolor : Outport
  wires:
  Switch2/1 -> RGBcolor/1
  on_off/1 -> Switch2/2
  Constant5/1 -> Switch2/3  "off"
  Constant9/1 -> Switch2/1  "on"

== system MCity_cs/VISUCasingLights_1_TrafficLightDoubleUS_7/conv_Orange ==
  on_off : Inport
  Constant2 : Constant  Value="[45 34 0 255  45 34 0 255  45 34 0 255  306 229 5 255]"
  Constant20 : Constant  Value=[32 25 5 255 64 48 5 255 64 54 5 255 0 0 0 255]
  Switch1 : Switch  Threshold=0.5
  RGBcolor : Outport
  wires:
  Constant20/1 -> Switch1/3  "off"
  Constant2/1 -> Switch1/1  "on"
  on_off/1 -> Switch1/2
  Switch1/1 -> RGBcolor/1

== system MCity_cs/VISUCasingLights_1_TrafficLightDoubleUS_7/conv_Red ==
  on_off : Inport
  Constant2 : Constant  Value="[45 0 0 255  45 0 0 255  45 0 0 255 306 30 30 255]"
  Constant20 : Constant  Value=[32 5 5 255 64 5 5 255 64 5 5 255 0 0 0 255]
  Switch1 : Switch  Threshold=0.5
  RGBcolor : Outport
  wires:
  Constant20/1 -> Switch1/3  "off"
  Constant2/1 -> Switch1/1  "on"
  on_off/1 -> Switch1/2
  Switch1/1 -> RGBcolor/1

== system MCity_cs/VISUCasingLights_1_TrafficLightDoubleUS_7/visu_CasingGreen ==
  Y : Inport
  Assignment : Assignment  IndexMode=Zero-based  SampleTime=TimeStep  IndexOptions=Starting index (dialog)  Indices=PortIndex  OutputSizes=[1 1]
  Data Store Read : DataStoreRead  DataStoreName=SimCoreActuators  SampleTime=TimeStep
  Data Store Write : DataStoreWrite  DataStoreName=SimCoreActuators
  wires:
  Assignment/1 -> Data Store Write/1
  Data Store Read/1 -> Assignment/1
  Y/1 -> Assignment/2

== system MCity_cs/VISUCasingLights_1_TrafficLightDoubleUS_7/visu_CasingOrange ==
  Y : Inport
  Assignment : Assignment  IndexMode=Zero-based  SampleTime=TimeStep  IndexOptions=Starting index (dialog)  Indices=PortIndex  OutputSizes=[1 1]
  Data Store Read : DataStoreRead  DataStoreName=SimCoreActuators  SampleTime=TimeStep
  Data Store Write : DataStoreWrite  DataStoreName=SimCoreActuators
  wires:
  Assignment/1 -> Data Store Write/1
  Data Store Read/1 -> Assignment/1
  Y/1 -> Assignment/2

== system MCity_cs/VISUCasingLights_1_TrafficLightDoubleUS_7/visu_CasingRed ==
  Y : Inport
  Assignment : Assignment  IndexMode=Zero-based  SampleTime=TimeStep  IndexOptions=Starting index (dialog)  Indices=PortIndex  OutputSizes=[1 1]
  Data Store Read : DataStoreRead  DataStoreName=SimCoreActuators  SampleTime=TimeStep
  Data Store Write : DataStoreWrite  DataStoreName=SimCoreActuators
  wires:
  Assignment/1 -> Data Store Write/1
  Data Store Read/1 -> Assignment/1
  Y/1 -> Assignment/2

== system MCity_cs/VISUCasingLights_1_TrafficLightDoubleUS_8/conv_Green ==
  on_off : Inport
  Constant5 : Constant  Value=[5 32 25 255 0 64 50 255 0 64 50 255 0 0 0 255]
  Constant9 : Constant  Value="[0 45 34 255  0 45 34 255  0 45 34 255  30 306 240 255]"
  Switch2 : Switch  Threshold=0.5
  RGBcolor : Outport
  wires:
  Switch2/1 -> RGBcolor/1
  on_off/1 -> Switch2/2
  Constant5/1 -> Switch2/3  "off"
  Constant9/1 -> Switch2/1  "on"

== system MCity_cs/VISUCasingLights_1_TrafficLightDoubleUS_8/conv_Orange ==
  on_off : Inport
  Constant2 : Constant  Value="[45 34 0 255  45 34 0 255  45 34 0 255  306 229 5 255]"
  Constant20 : Constant  Value=[32 25 5 255 64 48 5 255 64 54 5 255 0 0 0 255]
  Switch1 : Switch  Threshold=0.5
  RGBcolor : Outport
  wires:
  Constant20/1 -> Switch1/3  "off"
  Constant2/1 -> Switch1/1  "on"
  on_off/1 -> Switch1/2
  Switch1/1 -> RGBcolor/1

== system MCity_cs/VISUCasingLights_1_TrafficLightDoubleUS_8/conv_Red ==
  on_off : Inport
  Constant2 : Constant  Value="[45 0 0 255  45 0 0 255  45 0 0 255 306 30 30 255]"
  Constant20 : Constant  Value=[32 5 5 255 64 5 5 255 64 5 5 255 0 0 0 255]
  Switch1 : Switch  Threshold=0.5
  RGBcolor : Outport
  wires:
  Constant20/1 -> Switch1/3  "off"
  Constant2/1 -> Switch1/1  "on"
  on_off/1 -> Switch1/2
  Switch1/1 -> RGBcolor/1

== system MCity_cs/VISUCasingLights_1_TrafficLightDoubleUS_8/visu_CasingGreen ==
  Y : Inport
  Assignment : Assignment  IndexMode=Zero-based  SampleTime=TimeStep  IndexOptions=Starting index (dialog)  Indices=PortIndex  OutputSizes=[1 1]
  Data Store Read : DataStoreRead  DataStoreName=SimCoreActuators  SampleTime=TimeStep
  Data Store Write : DataStoreWrite  DataStoreName=SimCoreActuators
  wires:
  Assignment/1 -> Data Store Write/1
  Data Store Read/1 -> Assignment/1
  Y/1 -> Assignment/2

== system MCity_cs/VISUCasingLights_1_TrafficLightDoubleUS_8/visu_CasingOrange ==
  Y : Inport
  Assignment : Assignment  IndexMode=Zero-based  SampleTime=TimeStep  IndexOptions=Starting index (dialog)  Indices=PortIndex  OutputSizes=[1 1]
  Data Store Read : DataStoreRead  DataStoreName=SimCoreActuators  SampleTime=TimeStep
  Data Store Write : DataStoreWrite  DataStoreName=SimCoreActuators
  wires:
  Assignment/1 -> Data Store Write/1
  Data Store Read/1 -> Assignment/1
  Y/1 -> Assignment/2

== system MCity_cs/VISUCasingLights_1_TrafficLightDoubleUS_8/visu_CasingRed ==
  Y : Inport
  Assignment : Assignment  IndexMode=Zero-based  SampleTime=TimeStep  IndexOptions=Starting index (dialog)  Indices=PortIndex  OutputSizes=[1 1]
  Data Store Read : DataStoreRead  DataStoreName=SimCoreActuators  SampleTime=TimeStep
  Data Store Write : DataStoreWrite  DataStoreName=SimCoreActuators
  wires:
  Assignment/1 -> Data Store Write/1
  Data Store Read/1 -> Assignment/1
  Y/1 -> Assignment/2

== system MCity_cs/VISUCasingLights_1_TrafficLightDoubleUS_9/conv_Green ==
  on_off : Inport
  Constant5 : Constant  Value=[5 32 25 255 0 64 50 255 0 64 50 255 0 0 0 255]
  Constant9 : Constant  Value="[0 45 34 255  0 45 34 255  0 45 34 255  30 306 240 255]"
  Switch2 : Switch  Threshold=0.5
  RGBcolor : Outport
  wires:
  Switch2/1 -> RGBcolor/1
  on_off/1 -> Switch2/2
  Constant5/1 -> Switch2/3  "off"
  Constant9/1 -> Switch2/1  "on"

== system MCity_cs/VISUCasingLights_1_TrafficLightDoubleUS_9/conv_Orange ==
  on_off : Inport
  Constant2 : Constant  Value="[45 34 0 255  45 34 0 255  45 34 0 255  306 229 5 255]"
  Constant20 : Constant  Value=[32 25 5 255 64 48 5 255 64 54 5 255 0 0 0 255]
  Switch1 : Switch  Threshold=0.5
  RGBcolor : Outport
  wires:
  Constant20/1 -> Switch1/3  "off"
  Constant2/1 -> Switch1/1  "on"
  on_off/1 -> Switch1/2
  Switch1/1 -> RGBcolor/1

== system MCity_cs/VISUCasingLights_1_TrafficLightDoubleUS_9/conv_Red ==
  on_off : Inport
  Constant2 : Constant  Value="[45 0 0 255  45 0 0 255  45 0 0 255 306 30 30 255]"
  Constant20 : Constant  Value=[32 5 5 255 64 5 5 255 64 5 5 255 0 0 0 255]
  Switch1 : Switch  Threshold=0.5
  RGBcolor : Outport
  wires:
  Constant20/1 -> Switch1/3  "off"
  Constant2/1 -> Switch1/1  "on"
  on_off/1 -> Switch1/2
  Switch1/1 -> RGBcolor/1

== system MCity_cs/VISUCasingLights_1_TrafficLightDoubleUS_9/visu_CasingGreen ==
  Y : Inport
  Assignment : Assignment  IndexMode=Zero-based  SampleTime=TimeStep  IndexOptions=Starting index (dialog)  Indices=PortIndex  OutputSizes=[1 1]
  Data Store Read : DataStoreRead  DataStoreName=SimCoreActuators  SampleTime=TimeStep
  Data Store Write : DataStoreWrite  DataStoreName=SimCoreActuators
  wires:
  Assignment/1 -> Data Store Write/1
  Data Store Read/1 -> Assignment/1
  Y/1 -> Assignment/2

== system MCity_cs/VISUCasingLights_1_TrafficLightDoubleUS_9/visu_CasingOrange ==
  Y : Inport
  Assignment : Assignment  IndexMode=Zero-based  SampleTime=TimeStep  IndexOptions=Starting index (dialog)  Indices=PortIndex  OutputSizes=[1 1]
  Data Store Read : DataStoreRead  DataStoreName=SimCoreActuators  SampleTime=TimeStep
  Data Store Write : DataStoreWrite  DataStoreName=SimCoreActuators
  wires:
  Assignment/1 -> Data Store Write/1
  Data Store Read/1 -> Assignment/1
  Y/1 -> Assignment/2

== system MCity_cs/VISUCasingLights_1_TrafficLightDoubleUS_9/visu_CasingRed ==
  Y : Inport
  Assignment : Assignment  IndexMode=Zero-based  SampleTime=TimeStep  IndexOptions=Starting index (dialog)  Indices=PortIndex  OutputSizes=[1 1]
  Data Store Read : DataStoreRead  DataStoreName=SimCoreActuators  SampleTime=TimeStep
  Data Store Write : DataStoreWrite  DataStoreName=SimCoreActuators
  wires:
  Assignment/1 -> Data Store Write/1
  Data Store Read/1 -> Assignment/1
  Y/1 -> Assignment/2

== system MCity_cs/VISUCasingLights_2_TrafficLightDoubleUS_1/conv_Green ==
  on_off : Inport
  Constant5 : Constant  Value=[5 32 25 255 0 64 50 255 0 64 50 255 0 0 0 255]
  Constant9 : Constant  Value="[0 45 34 255  0 45 34 255  0 45 34 255  30 306 240 255]"
  Switch2 : Switch  Threshold=0.5
  RGBcolor : Outport
  wires:
  Switch2/1 -> RGBcolor/1
  on_off/1 -> Switch2/2
  Constant5/1 -> Switch2/3  "off"
  Constant9/1 -> Switch2/1  "on"

== system MCity_cs/VISUCasingLights_2_TrafficLightDoubleUS_1/conv_Orange ==
  on_off : Inport
  Constant2 : Constant  Value="[45 34 0 255  45 34 0 255  45 34 0 255  306 229 5 255]"
  Constant20 : Constant  Value=[32 25 5 255 64 48 5 255 64 54 5 255 0 0 0 255]
  Switch1 : Switch  Threshold=0.5
  RGBcolor : Outport
  wires:
  Constant20/1 -> Switch1/3  "off"
  Constant2/1 -> Switch1/1  "on"
  on_off/1 -> Switch1/2
  Switch1/1 -> RGBcolor/1

== system MCity_cs/VISUCasingLights_2_TrafficLightDoubleUS_1/conv_Red ==
  on_off : Inport
  Constant2 : Constant  Value="[45 0 0 255  45 0 0 255  45 0 0 255 306 30 30 255]"
  Constant20 : Constant  Value=[32 5 5 255 64 5 5 255 64 5 5 255 0 0 0 255]
  Switch1 : Switch  Threshold=0.5
  RGBcolor : Outport
  wires:
  Constant20/1 -> Switch1/3  "off"
  Constant2/1 -> Switch1/1  "on"
  on_off/1 -> Switch1/2
  Switch1/1 -> RGBcolor/1

== system MCity_cs/VISUCasingLights_2_TrafficLightDoubleUS_1/visu_CasingGreen ==
  Y : Inport
  Assignment : Assignment  IndexMode=Zero-based  SampleTime=TimeStep  IndexOptions=Starting index (dialog)  Indices=PortIndex  OutputSizes=[1 1]
  Data Store Read : DataStoreRead  DataStoreName=SimCoreActuators  SampleTime=TimeStep
  Data Store Write : DataStoreWrite  DataStoreName=SimCoreActuators
  wires:
  Assignment/1 -> Data Store Write/1
  Data Store Read/1 -> Assignment/1
  Y/1 -> Assignment/2

== system MCity_cs/VISUCasingLights_2_TrafficLightDoubleUS_1/visu_CasingOrange ==
  Y : Inport
  Assignment : Assignment  IndexMode=Zero-based  SampleTime=TimeStep  IndexOptions=Starting index (dialog)  Indices=PortIndex  OutputSizes=[1 1]
  Data Store Read : DataStoreRead  DataStoreName=SimCoreActuators  SampleTime=TimeStep
  Data Store Write : DataStoreWrite  DataStoreName=SimCoreActuators
  wires:
  Assignment/1 -> Data Store Write/1
  Data Store Read/1 -> Assignment/1
  Y/1 -> Assignment/2

== system MCity_cs/VISUCasingLights_2_TrafficLightDoubleUS_1/visu_CasingRed ==
  Y : Inport
  Assignment : Assignment  IndexMode=Zero-based  SampleTime=TimeStep  IndexOptions=Starting index (dialog)  Indices=PortIndex  OutputSizes=[1 1]
  Data Store Read : DataStoreRead  DataStoreName=SimCoreActuators  SampleTime=TimeStep
  Data Store Write : DataStoreWrite  DataStoreName=SimCoreActuators
  wires:
  Assignment/1 -> Data Store Write/1
  Data Store Read/1 -> Assignment/1
  Y/1 -> Assignment/2

== system MCity_cs/VISUCasingLights_2_TrafficLightDoubleUS_10/conv_Green ==
  on_off : Inport
  Constant5 : Constant  Value=[5 32 25 255 0 64 50 255 0 64 50 255 0 0 0 255]
  Constant9 : Constant  Value="[0 45 34 255  0 45 34 255  0 45 34 255  30 306 240 255]"
  Switch2 : Switch  Threshold=0.5
  RGBcolor : Outport
  wires:
  Switch2/1 -> RGBcolor/1
  on_off/1 -> Switch2/2
  Constant5/1 -> Switch2/3  "off"
  Constant9/1 -> Switch2/1  "on"

== system MCity_cs/VISUCasingLights_2_TrafficLightDoubleUS_10/conv_Orange ==
  on_off : Inport
  Constant2 : Constant  Value="[45 34 0 255  45 34 0 255  45 34 0 255  306 229 5 255]"
  Constant20 : Constant  Value=[32 25 5 255 64 48 5 255 64 54 5 255 0 0 0 255]
  Switch1 : Switch  Threshold=0.5
  RGBcolor : Outport
  wires:
  Constant20/1 -> Switch1/3  "off"
  Constant2/1 -> Switch1/1  "on"
  on_off/1 -> Switch1/2
  Switch1/1 -> RGBcolor/1

== system MCity_cs/VISUCasingLights_2_TrafficLightDoubleUS_10/conv_Red ==
  on_off : Inport
  Constant2 : Constant  Value="[45 0 0 255  45 0 0 255  45 0 0 255 306 30 30 255]"
  Constant20 : Constant  Value=[32 5 5 255 64 5 5 255 64 5 5 255 0 0 0 255]
  Switch1 : Switch  Threshold=0.5
  RGBcolor : Outport
  wires:
  Constant20/1 -> Switch1/3  "off"
  Constant2/1 -> Switch1/1  "on"
  on_off/1 -> Switch1/2
  Switch1/1 -> RGBcolor/1

== system MCity_cs/VISUCasingLights_2_TrafficLightDoubleUS_10/visu_CasingGreen ==
  Y : Inport
  Assignment : Assignment  IndexMode=Zero-based  SampleTime=TimeStep  IndexOptions=Starting index (dialog)  Indices=PortIndex  OutputSizes=[1 1]
  Data Store Read : DataStoreRead  DataStoreName=SimCoreActuators  SampleTime=TimeStep
  Data Store Write : DataStoreWrite  DataStoreName=SimCoreActuators
  wires:
  Assignment/1 -> Data Store Write/1
  Data Store Read/1 -> Assignment/1
  Y/1 -> Assignment/2

== system MCity_cs/VISUCasingLights_2_TrafficLightDoubleUS_10/visu_CasingOrange ==
  Y : Inport
  Assignment : Assignment  IndexMode=Zero-based  SampleTime=TimeStep  IndexOptions=Starting index (dialog)  Indices=PortIndex  OutputSizes=[1 1]
  Data Store Read : DataStoreRead  DataStoreName=SimCoreActuators  SampleTime=TimeStep
  Data Store Write : DataStoreWrite  DataStoreName=SimCoreActuators
  wires:
  Assignment/1 -> Data Store Write/1
  Data Store Read/1 -> Assignment/1
  Y/1 -> Assignment/2

== system MCity_cs/VISUCasingLights_2_TrafficLightDoubleUS_10/visu_CasingRed ==
  Y : Inport
  Assignment : Assignment  IndexMode=Zero-based  SampleTime=TimeStep  IndexOptions=Starting index (dialog)  Indices=PortIndex  OutputSizes=[1 1]
  Data Store Read : DataStoreRead  DataStoreName=SimCoreActuators  SampleTime=TimeStep
  Data Store Write : DataStoreWrite  DataStoreName=SimCoreActuators
  wires:
  Assignment/1 -> Data Store Write/1
  Data Store Read/1 -> Assignment/1
  Y/1 -> Assignment/2

== system MCity_cs/VISUCasingLights_2_TrafficLightDoubleUS_2/conv_Green ==
  on_off : Inport
  Constant5 : Constant  Value=[5 32 25 255 0 64 50 255 0 64 50 255 0 0 0 255]
  Constant9 : Constant  Value="[0 45 34 255  0 45 34 255  0 45 34 255  30 306 240 255]"
  Switch2 : Switch  Threshold=0.5
  RGBcolor : Outport
  wires:
  Switch2/1 -> RGBcolor/1
  on_off/1 -> Switch2/2
  Constant5/1 -> Switch2/3  "off"
  Constant9/1 -> Switch2/1  "on"

== system MCity_cs/VISUCasingLights_2_TrafficLightDoubleUS_2/conv_Orange ==
  on_off : Inport
  Constant2 : Constant  Value="[45 34 0 255  45 34 0 255  45 34 0 255  306 229 5 255]"
  Constant20 : Constant  Value=[32 25 5 255 64 48 5 255 64 54 5 255 0 0 0 255]
  Switch1 : Switch  Threshold=0.5
  RGBcolor : Outport
  wires:
  Constant20/1 -> Switch1/3  "off"
  Constant2/1 -> Switch1/1  "on"
  on_off/1 -> Switch1/2
  Switch1/1 -> RGBcolor/1

== system MCity_cs/VISUCasingLights_2_TrafficLightDoubleUS_2/conv_Red ==
  on_off : Inport
  Constant2 : Constant  Value="[45 0 0 255  45 0 0 255  45 0 0 255 306 30 30 255]"
  Constant20 : Constant  Value=[32 5 5 255 64 5 5 255 64 5 5 255 0 0 0 255]
  Switch1 : Switch  Threshold=0.5
  RGBcolor : Outport
  wires:
  Constant20/1 -> Switch1/3  "off"
  Constant2/1 -> Switch1/1  "on"
  on_off/1 -> Switch1/2
  Switch1/1 -> RGBcolor/1
